simulink model "Projeto"  (R2020a)
settings: Solver=VariableStepAuto  StartTime=0.0  StopTime=10  RelTol=1e-3
values from neighbouring files (symbols this model uses):
  A = [0 1 0;(k*(x3^2))/(m*(x1^3)) 0 (-2*k*x3)/(m*(x1^2));0 (2*k*x3)/(L*(x1^2)) -R/L]    [ProjetoCD.m]
  B = [0;0;1/L]    [ProjetoCD.m]
  C = [1 0 0]    [ProjetoCD.m]
  F = [s1f1 s1f2 s1f3]    [ProjetoCD.m]
  fa = double(s1fa)    [ProjetoCD.m]
  L = [s1l1;s1l2;s1l3]    [ProjetoCD.m]
  T = 0.01    [ProjetoCD.m]
  x1 = 0.012    [ProjetoCD.m]
  x2 = 0    [ProjetoCD.m]
  x3 = x1*sqrt(g*m/k)    [ProjetoCD.m]
undefined symbols (not defined in the file or in its folder): G, H
libraries: simulink x1
settings Model: Creator=joaov  LastModifiedBy=joaov

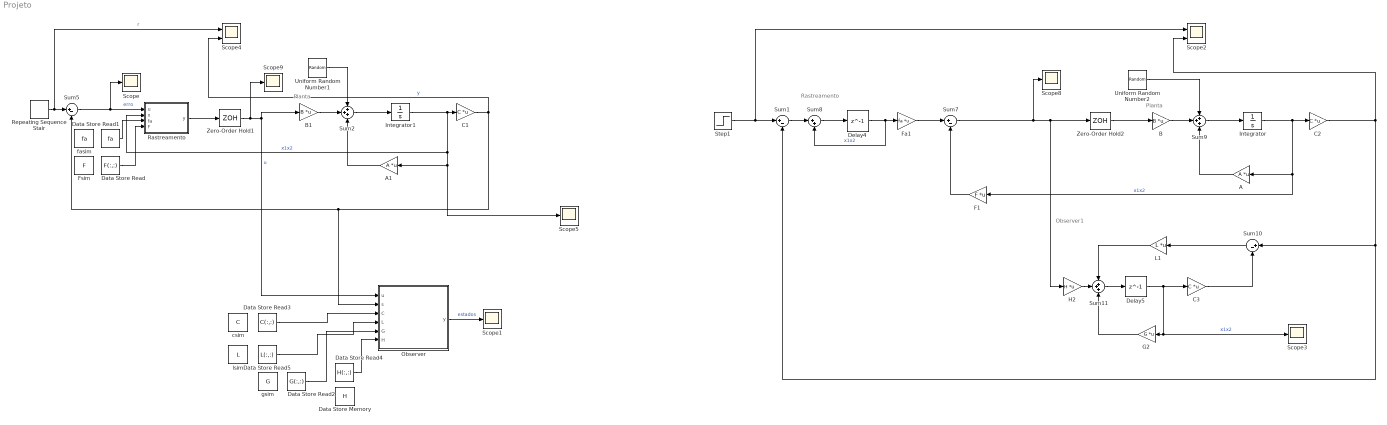
== system Projeto ==
  note: Rastreamento
  note: Observer1
  note: Planta
  note: Planta
  A : Gain  Gain=A  Multiplication=Matrix(K*u)
  A1 : Gain  Gain=A  Multiplication=Matrix(K*u)
  B : Gain  Gain=B  Multiplication=Matrix(K*u)
  B1 : Gain  Gain=B  Multiplication=Matrix(K*u)
  C1 : Gain  Gain=C  Multiplication=Matrix(K*u)
  C2 : Gain  Gain=C  Multiplication=Matrix(K*u)
  C3 : Gain  Gain=C  Multiplication=Matrix(K*u)
  Data Store Memory : DataStoreMemory  DataStoreName=H  ReadBeforeWriteMsg=warning  WriteAfterWriteMsg=warning  WriteAfterReadMsg=warning  InitialValue=H  ShareAcrossModelInstances=on  VectorParams1D=off  ShowAdditionalParam=off
  Data Store Read : DataStoreRead  DataStoreName=F  SampleTime=T  DataStoreElements=F(:,:)
  Data Store Read1 : DataStoreRead  DataStoreName=fa  SampleTime=T  DataStoreElements=fa
  Data Store Read2 : DataStoreRead  DataStoreName=G  SampleTime=T  DataStoreElements=G(:,:)
  Data Store Read3 : DataStoreRead  DataStoreName=C  SampleTime=T  DataStoreElements=C(:,:)
  Data Store Read4 : DataStoreRead  DataStoreName=H  SampleTime=T  DataStoreElements=H(:,:)
  Data Store Read5 : DataStoreRead  DataStoreName=L  SampleTime=T  DataStoreElements=L(:,:)
  Delay4 : Delay  DelayLength=1  InitialCondition=0  SampleTime=T
  Delay5 : Delay  DelayLength=1  InitialCondition=0  SampleTime=T
  F1 : Gain  Gain=F  Multiplication=Matrix(K*u)
  Fa1 : Gain  Gain=fa  Multiplication=Matrix(K*u)
  Fsim : DataStoreMemory  DataStoreName=F  ReadBeforeWriteMsg=warning  WriteAfterWriteMsg=warning  WriteAfterReadMsg=warning  InitialValue=F  ShareAcrossModelInstances=on  VectorParams1D=off  ShowAdditionalParam=off
  G2 : Gain  Gain=G  Multiplication=Matrix(K*u)
  H2 : Gain  Gain=H  Multiplication=Matrix(K*u)
  Integrator : Integrator  InitialCondition=[0;0;0]
  Integrator1 : Integrator  InitialCondition=[x1;x2;x3]
  L1 : Gain  Gain=L  Multiplication=Matrix(K*u)
  Observer : MATLAB Function  TreatAsAtomicUnit=on
  Rastreamento : MATLAB Function  TreatAsAtomicUnit=on
  Repeating Sequence Stair : simulink/Sources/Repeating Sequence Stair  OutValues=[0.03 0.01 0.04 0.02 0.01].'  tsamp=1  OutMin=[]  OutMax=[]  OutDataTypeStr=double  OutputDataTypeScalingMode=double  OutDataType=fixdt(0,8)  ConRadixGroup=Best Precision: Vector-wise  OutScaling=2^-12
  Scope{,1,3,5,8..9} (6 alike) : Scope
  Scope2 : Scope  NumInputPorts=2
  Scope4 : Scope  NumInputPorts=2
  Step1 : Step  After=0.012  SampleTime=T
  Sum{1,5,7,10} (4 alike) : Sum  Inputs=|+-
  Sum11 : Sum  Inputs=+++
  Sum2 : Sum  Inputs=+++
  Sum8 : Sum  Inputs=|++
  Sum9 : Sum  Inputs=+++
  Uniform Random Number1 : UniformRandomNumber  Minimum=-0.003  Maximum=0.003  SampleTime=T
  Uniform Random Number2 : UniformRandomNumber  Minimum=-0.003  Maximum=0.003  SampleTime=T
  Zero-Order Hold1 : ZeroOrderHold  SampleTime=T
  Zero-Order Hold2 : ZeroOrderHold  SampleTime=T
  csim : DataStoreMemory  DataStoreName=C  ReadBeforeWriteMsg=warning  WriteAfterWriteMsg=warning  WriteAfterReadMsg=warning  InitialValue=C  ShareAcrossModelInstances=on  VectorParams1D=off  ShowAdditionalParam=off
  fasim : DataStoreMemory  DataStoreName=fa  ReadBeforeWriteMsg=warning  WriteAfterWriteMsg=warning  WriteAfterReadMsg=warning  InitialValue=fa  ShareAcrossModelInstances=on  VectorParams1D=off  ShowAdditionalParam=off
  gsim : DataStoreMemory  DataStoreName=G  ReadBeforeWriteMsg=warning  WriteAfterWriteMsg=warning  WriteAfterReadMsg=warning  InitialValue=G  ShareAcrossModelInstances=on  VectorParams1D=off  ShowAdditionalParam=off
  lsim : DataStoreMemory  DataStoreName=L  ReadBeforeWriteMsg=warning  WriteAfterWriteMsg=warning  WriteAfterReadMsg=warning  InitialValue=L  ShareAcrossModelInstances=on  VectorParams1D=off  ShowAdditionalParam=off
  wires:
  Step1/1 -> Scope2/1, Sum1/1
  Sum1/1 -> Sum8/1
  Delay4/1 -> Sum8/2, Fa1/1  "x1x2"
  F1/1 -> Sum7/2
  Sum8/1 -> Delay4/1
  Fa1/1 -> Sum7/1
  H2/1 -> Sum11/2
  C2/1 -> Scope2/2, Sum10/1, Sum1/2
  G2/1 -> Sum11/3
  C3/1 -> Sum10/2
  L1/1 -> Sum11/1
  Sum11/1 -> Delay5/1
  Delay5/1 -> C3/1, Scope3/1, G2/1  "x1x2"
  Sum10/1 -> L1/1
  Sum9/1 -> Integrator/1
  Sum7/1 -> Zero-Order Hold2/1, H2/1, Scope8/1
  A1/1 -> Sum2/3
  Sum2/1 -> Integrator1/1
  B1/1 -> Sum2/2
  Integrator1/1 -> Scope5/1, A1/1, Rastreamento/2(x), C1/1  "x1x2"
  C1/1 -> Scope4/2, Observer/2(s), Sum5/2  "y"
  Repeating Sequence Stair/1 -> Scope4/1, Sum5/1  "r"
  Rastreamento/1(y) -> Zero-Order Hold1/1
  Sum5/1 -> Rastreamento/1(u), Scope/1  "erro"
  Data Store Read1/1 -> Rastreamento/3(fa)
  Data Store Read/1 -> Rastreamento/4(F)
  Zero-Order Hold1/1 -> Scope9/1, Observer/1(u), B1/1  "u"
  Data Store Read2/1 -> Observer/5(G)
  Data Store Read5/1 -> Observer/4(L)
  Data Store Read3/1 -> Observer/3(C)
  A/1 -> Sum9/3
  B/1 -> Sum9/2
  Uniform Random Number2/1 -> Sum9/1
  Uniform Random Number1/1 -> Sum2/1
  Zero-Order Hold2/1 -> B/1
  Data Store Read4/1 -> Observer/6(H)
  Observer/1(y) -> Scope1/1  "estados"
  Integrator/1 -> F1/1, A/1, C2/1  "x1x2"

== matlab function Projeto/Observer ==
  settings: updateMethod=DISCRETE  sampleTime=T
  data: u input; y output; s input; C input; L input; G input; H input
function y = fcn(u,s,C,L,G,H)
persistent u_d y_d;
if isempty(u_d)
   u_d = cast(0, 'like', u);
end
if isempty(y_d)
   y_d = cast([0;0;0], 'like', [0;0;0]);
end
y =  (u_d*H)+ L*(s - C*y_d) + G*y_d;
u_d = u;
y_d = y;

== matlab function Projeto/Rastreamento ==
  settings: updateMethod=DISCRETE  sampleTime=T
  data: u input; y output; x input; fa input; F input
function y = fcn(u,x,fa,F)
 persistent u_d y_d;
 if isempty(u_d)
    u_d = cast(0, 'like', u);
 end
 if isempty(y_d)
    y_d = cast(0, 'like', u);
 end
 y2 = u_d + y_d;
 u_d = u;
 y_d = y2;
 y = (y2*fa) - (F*x);
